simulink model "busassignment_test"  (Simulink 8.4)
settings: Solver=VariableStepDiscrete  StartTime=0.0  StopTime=0  MaxStep=1  RelTol=1e-3
undefined symbols (not defined in the file or in its folder): a2, a3
settings Model: Creator=arnaud  LastModifiedBy=arnaud
settings DataIOCC: SaveFormat=Structure  SignalLoggingSaveFormat=Dataset
settings OptimizationCC: ExpressionDepthLimit=128
settings DebuggingCC: UnderspecifiedInitializationDetection=Simplified  MergeDetectMultiDrivingBlocksExec=error  FcnCallInpInsideContextMsg=EnableAllAsError  StateNameClashWarn=none
settings GRTTargetCC: CombineOutputUpdateFcns=on  GRTInterface=off

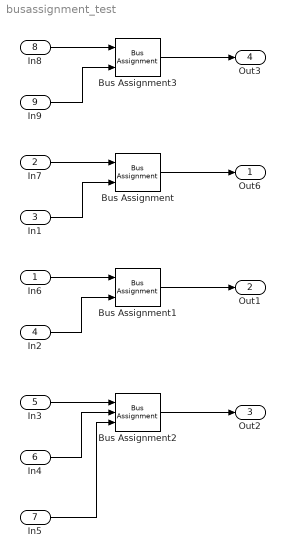
== system busassignment_test ==
  In6 : Inport  OutDataTypeStr=Bus: BusA  BusOutputAsStruct=on
  In7 : Inport  Port=2  OutDataTypeStr=Bus: BusUnif
  In1 : Inport  Port=3  OutDataTypeStr=double  PortDimensions=1
  In2 : Inport  Port=4  OutDataTypeStr=int16  PortDimensions=[2 3]
  In3 : Inport  Port=5  OutDataTypeStr=Bus: BusA  BusOutputAsStruct=on
  In4 : Inport  Port=6  OutDataTypeStr=boolean
  In5 : Inport  Port=7  OutDataTypeStr=double
  In8 : Inport  Port=8  OutDataTypeStr=Bus: BusUnif
  In9 : Inport  Port=9  OutDataTypeStr=double  PortDimensions=3
  Bus Assignment : BusAssignment  AssignedSignals=f
  Bus Assignment1 : BusAssignment  AssignedSignals=a1
  Bus Assignment2 : BusAssignment  AssignedSignals=a2,a3
  Bus Assignment3 : BusAssignment  AssignedSignals=f1
  Out6 : Outport
  Out1 : Outport  Port=2
  Out2 : Outport  Port=3
  Out3 : Outport  Port=4
  wires:
  In7/1 -> Bus Assignment/1
  In1/1 -> Bus Assignment/2
  Bus Assignment/1 -> Out6/1
  In6/1 -> Bus Assignment1/1
  In2/1 -> Bus Assignment1/2
  Bus Assignment1/1 -> Out1/1
  In3/1 -> Bus Assignment2/1
  In4/1 -> Bus Assignment2/2
  Bus Assignment2/1 -> Out2/1
  In5/1 -> Bus Assignment2/3
  In8/1 -> Bus Assignment3/1
  In9/1 -> Bus Assignment3/2
  Bus Assignment3/1 -> Out3/1
